simulink model "control"  (R2020b)
settings: Solver=VariableStepAuto  StartTime=0.0  StopTime=10.0  RelTol=1e-3
model workspace (MAT data in the model file):
  dt_planner = 0.01
undefined symbols (not defined in the file): DiscIntNeverNeededParam
settings Model: Creator=VVM  LastModifiedBy=VVM

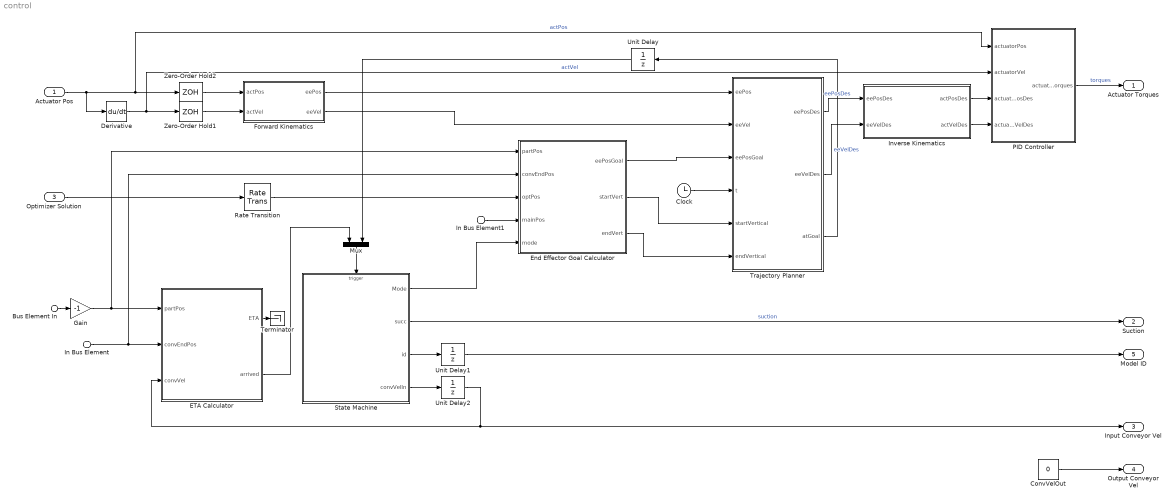
== system control ==
  Actuator Pos : Inport
  Bus Element In : Inport  Port=2  PortName=Camera Data  Element=model_position
  In Bus Element : Inport  Port=2  PortName=Camera Data  Element=beltEndPos
  In Bus Element1 : Inport  Port=2  PortName=Camera Data  Element=containerPos
  Optimizer Solution : Inport  Port=3
  Clock : Clock
  ConvVelOut : Constant  Value=0
  Derivative : Derivative  CoefficientInTFapproximation=0.0005
  ETA Calculator : MATLAB Function  TreatAsAtomicUnit=on
  End Effector Goal Calculator : MATLAB Function  TreatAsAtomicUnit=on
  Forward Kinematics : Subsystem
  Gain : Gain  Gain=-1
  Inverse Kinematics : Subsystem
  Mux : Mux  Inputs=2
  PID Controller : Subsystem  TreatAsAtomicUnit=on  mask(PID Controller){P=0.5, I=6, D=0.15}
  Rate Transition : RateTransition
  State Machine : Stateflow chart  TreatAsAtomicUnit=on
  Terminator : Terminator
  Trajectory Planner : MATLAB Function  TreatAsAtomicUnit=on
  Unit Delay : UnitDelay  SampleTime=-1  HasFrameUpgradeWarning=on
  Unit Delay1 : UnitDelay  InitialCondition=1  SampleTime=-1  HasFrameUpgradeWarning=on
  Unit Delay2 : UnitDelay  InitialCondition=1  SampleTime=-1  HasFrameUpgradeWarning=on
  Zero-Order Hold1 : ZeroOrderHold  SampleTime=-1
  Zero-Order Hold2 : ZeroOrderHold  SampleTime=-1
  Actuator Torques : Outport
  Suction : Outport  Port=2
  Input Conveyor Vel : Outport  Port=3
  Output Conveyor Vel : Outport  Port=4
  Model ID : Outport  Port=5
  wires:
  Optimizer Solution/1 -> Rate Transition/1
  State Machine/3(id) -> Unit Delay1/1
  Gain/1 -> End Effector Goal Calculator/1(partPos), ETA Calculator/1(partPos)
  ETA Calculator/1(ETA) -> Terminator/1
  Trajectory Planner/3(atGoal) -> Unit Delay/1
  Unit Delay1/1 -> Model ID/1
  Rate Transition/1 -> End Effector Goal Calculator/3(optPos)
  State Machine/2(succ) -> Suction/1  "suction"
  State Machine/1(Mode) -> End Effector Goal Calculator/5(mode)
  End Effector Goal Calculator/3(endVert) -> Trajectory Planner/6(endVertical)
  End Effector Goal Calculator/1(eePosGoal) -> Trajectory Planner/3(eePosGoal)
  End Effector Goal Calculator/2(startVert) -> Trajectory Planner/5(startVertical)
  Unit Delay2/1 -> Input Conveyor Vel/1, ETA Calculator/3(convVel)
  Mux/1 -> State Machine/Trigger
  Actuator Pos/1 -> Zero-Order Hold2/1, PID Controller/1(actuatorPos), Derivative/1  "actPos"
  State Machine/4(convVelIn) -> Unit Delay2/1
  Zero-Order Hold1/1 -> Forward Kinematics/2(actVel)
  Zero-Order Hold2/1 -> Forward Kinematics/1(actPos)
  Derivative/1 -> Zero-Order Hold1/1, PID Controller/2(actuatorVel)  "actVel"
  Inverse Kinematics/2(actVelDes) -> PID Controller/4(actuatorVelDes)
  Inverse Kinematics/1(actPosDes) -> PID Controller/3(actuatorPosDes)
  Unit Delay/1 -> Mux/2
  Trajectory Planner/1(eePosDes) -> Inverse Kinematics/1(eePosDes)  "eePosDes"
  ConvVelOut/1 -> Output Conveyor Vel/1
  In Bus Element/1 -> End Effector Goal Calculator/2(convEndPos), ETA Calculator/2(convEndPos)
  Forward Kinematics/2(eeVel) -> Trajectory Planner/2(eeVel)
  Clock/1 -> Trajectory Planner/4(t)
  Forward Kinematics/1(eePos) -> Trajectory Planner/1(eePos)
  PID Controller/1(actuatorTorques) -> Actuator Torques/1  "torques"
  Trajectory Planner/2(eeVelDes) -> Inverse Kinematics/2(eeVelDes)  "eeVelDes"
  ETA Calculator/2(arrived) -> Mux/1
  In Bus Element1/1 -> End Effector Goal Calculator/4(mainPos)
  Bus Element In/1 -> Gain/1

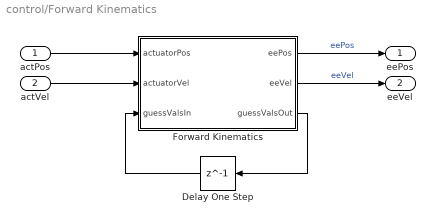
== system control/Forward Kinematics ==
  actPos : Inport
  actVel : Inport  Port=2
  Delay One Step : Delay  DelayLength=1
  Forward Kinematics : MATLAB Function  TreatAsAtomicUnit=on
  eePos : Outport
  eeVel : Outport  Port=2
  wires:
  Delay One Step/1 -> Forward Kinematics/3(guessValsIn)
  Forward Kinematics/3(guessValsOut) -> Delay One Step/1
  actPos/1 -> Forward Kinematics/1(actuatorPos)
  actVel/1 -> Forward Kinematics/2(actuatorVel)
  Forward Kinematics/1(eePos) -> eePos/1  "eePos"
  Forward Kinematics/2(eeVel) -> eeVel/1  "eeVel"

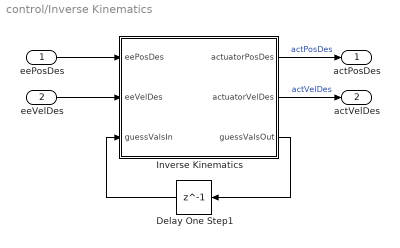
== system control/Inverse Kinematics ==
  eePosDes : Inport
  eeVelDes : Inport  Port=2
  Delay One Step1 : Delay  DelayLength=1
  Inverse Kinematics : MATLAB Function  TreatAsAtomicUnit=on
  actPosDes : Outport
  actVelDes : Outport  Port=2
  wires:
  Delay One Step1/1 -> Inverse Kinematics/3(guessValsIn)
  Inverse Kinematics/3(guessValsOut) -> Delay One Step1/1
  Inverse Kinematics/2(actuatorVelDes) -> actVelDes/1  "actVelDes"
  Inverse Kinematics/1(actuatorPosDes) -> actPosDes/1  "actPosDes"
  eeVelDes/1 -> Inverse Kinematics/2(eeVelDes)
  eePosDes/1 -> Inverse Kinematics/1(eePosDes)

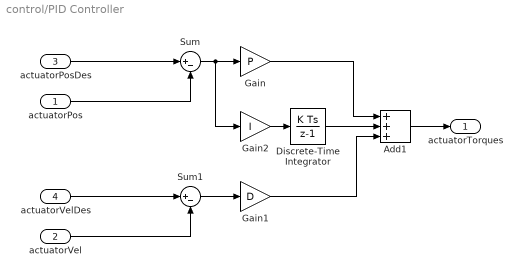
== system control/PID Controller ==
  actuatorPos : Inport
  actuatorVel : Inport  Port=2
  actuatorPosDes : Inport  Port=3
  actuatorVelDes : Inport  Port=4
  Add1 : Sum  Inputs=+++
  Discrete-Time Integrator : DiscreteIntegrator  gainval=1  SampleTime=-1  ICPrevOutput=DiscIntNeverNeededParam  ICPrevScaledInput=DiscIntNeverNeededParam
  Gain : Gain  Gain=P
  Gain1 : Gain  Gain=D
  Gain2 : Gain  Gain=I
  Sum : Sum  Inputs=|+-
  Sum1 : Sum  Inputs=|+-
  actuatorTorques : Outport
  wires:
  actuatorPosDes/1 -> Sum/1
  actuatorPos/1 -> Sum/2
  actuatorVel/1 -> Sum1/2
  Sum/1 -> Gain2/1, Gain/1
  Sum1/1 -> Gain1/1
  Gain/1 -> Add1/1
  Gain1/1 -> Add1/3
  Discrete-Time Integrator/1 -> Add1/2
  Gain2/1 -> Discrete-Time Integrator/1
  Add1/1 -> actuatorTorques/1
  actuatorVelDes/1 -> Sum1/1

== stateflow chart control/State Machine ==
  settings: executeAtInitialization=1
  state Hover
  state Grab
    entry:
    convVelIn = 0;
    exit:
    convVelIn = 1;
  state Retract2
  state Retract1
  state Drop
  note: Wait for object
      | to stabilize
  Hover -> Grab : arrived
  Grab -> Retract2 : atGoal
      | {succ = 1;}
  Retract1 -> Hover : atGoal
  Retract2 -> Drop : atGoal
  (default) -> Retract1
  (junction 406) -> Retract1 : after(15,msec)
      | {succ = 0; id = id + 1;}
  Drop -> (junction 406) : atGoal
  data: Mode output Enum: State; succ output; id output =1; convVelIn output =1
  events: arrived input RISING_EDGE_EVENT; atGoal input RISING_EDGE_EVENT

== matlab function control/Forward Kinematics/Forward Kinematics ==
  settings: updateMethod=DISCRETE  sampleTime=0.01
  data: actuatorPos input size=3; eePos output size=3; actuatorVel input size=3; guessValsIn input size=3; eeVel output; guessValsOut output size=3
function [eePos, eeVel, guessValsOut] = FK(actuatorPos, actuatorVel, guessValsIn)
% Wrapper around sm_pick_and_place_fk.m, which creates a persistent
% KinematicsSolver object for the forwards kinematics problem and then
% solves it.

coder.extrinsic('fk_solver');
persistent init
if isempty(init)
    init = true;
    eePos = zeros(3,1);
    eeVel = zeros(3,1);
    guessValsOut = zeros(3,1);
    status = 1;
end
[eePos, eeVel, guessValsOut, status] = fk_solver(actuatorPos, actuatorVel, guessValsIn);
if status ~= 1
    error('404 solution not found. Forward solve failed.')
end

== matlab function control/Inverse Kinematics/Inverse Kinematics ==
  settings: updateMethod=DISCRETE  sampleTime=0.01
  data: eePosDes input size=3; actuatorPosDes output size=3; eeVelDes input size=3; guessValsIn input size=3; actuatorVelDes output size=3; guessValsOut output size=3
function [actuatorPosDes, actuatorVelDes, guessValsOut] = IK(eePosDes, eeVelDes, guessValsIn)
% Wrapper around sm_pick_and_place_ik.m, which creates a persistent
% KinematicsSolver object for the inverse kinematics problem and then
% solves it.

coder.extrinsic('ik_solver');
persistent init
if isempty(init)
    init = true;
    actuatorPosDes = zeros(3,1);
    actuatorVelDes = zeros(3,1);
    guessValsOut = zeros(3,1);
    status = 1;
end
[actuatorPosDes, actuatorVelDes, guessValsOut, status] = ik_solver(eePosDes, eeVelDes, guessValsIn);
if status ~= 1
    error("Mathworks but your math doesn't. Inverse solve failed.");
end

== matlab function control/Trajectory Planner ==
  settings: updateMethod=DISCRETE
  data: eePos input size=3; eeVel input size=3; eePosGoal input size=3; eePosDes output size=3; t input size=1; startVertical input size=1; endVertical input size=1; eeVelDes output size=3; atGoal output
function [eePosDes, eeVelDes, atGoal] = gotoPosition(eePos, eeVel, eePosGoal, t, startVertical, endVertical)
% High-level function to go to a goal position.  Returns the desired
% position and and velocity at current time along the trajectory to a goal
% position. The time to goal along the trajectory is always set to 0.2
% seconds. startVertical and endVertical indicate whether the curve defined
% by the trajectory should begin and/or end vertically (i.e., the end
% effector should move straight up or down when starting or ending its
% motion).  It always assumed that the initial and final velocities and
% accelerations along the trajectory are zero.  Thus, the goal velocity is
% always zero. If the current position and velocity are sufficiently close
% to the goal position and velocity, 'done' is true.

persistent plan
if isempty(plan)
    plan = true;
end

if startVertical
    startDirectionGoal = [0;0;-0.2];
else
    startDirectionGoal = eeVel;
end
if endVertical
    endDirectionGoal = [0;0;0.2];
else
    endDirectionGoal = [0;0;0];
end
timeToGoal = 0.3;
[eePosDes, eeVelDes, atGoal] = gotoGoal(...
    plan, ...
    t, timeToGoal, ...
    eePos, eeVel, ...
    eePosGoal, startDirectionGoal, endDirectionGoal);
plan = atGoal;
end

function p = getPoly5(t0,tf,x0,v0,a0,xf,vf,af)
% Compute the 5th order polynomial 
% 
% poly(t) = a*t^5 + b*t^4 + c*t^3 + d*t^2 + e*t + f
%
% such that
%
% p(t0) = x0; p(tf) = xf
% p'(t0) = v0; p'(tf) = vf
% p''(to) = a0; p''(tf) = af
%
% Returns the coeffecient vector p = [a b c d e f]

A = [t0^5    t0^4    t0^3   t0^2 t0 1;
     5*t0^4  4*t0^3  3*t0^2 2*t0 1  0;
     20*t0^3 12*t0^2 6*t0   2    0  0;
     tf^5    tf^4    tf^3   tf^2 tf 1;
     5*tf^4  4*tf^3  3*tf^2 2*tf 1  0;
     20*tf^3 12*tf^2 6*tf   2    0  0];
b = [x0 v0 a0 xf vf af]';
p = A\b;
end

function p = getPoly3(t0,tf,x0,v0,xf,vf)
% Compute the 3rd order polynomial 
% 
% poly(t) = a*t^3 + b*t^2 + c*t + d
%
% such that
%
% p(t0) = x0; p(tf) = xf
% p'(t0) = v0; p'(tf) = vf
%
% Returns the coeffecient vector p = [a b c d]

A = [t0^3   t0^2 t0 1;
     3*t0^2 2*t0 1  0;
     tf^3   tf^2 tf 1;
     3*tf^2 2*tf 1  0];
b = [x0 v0 xf vf]';
p = A\b;
end

function [eePosDes, eeVelDes, atGoal] = gotoGoal(...
    plan, ...
    t, timeToGoal, ...
    eePos, eeVel, ...
    eePosGoal, startDirectionGoal, endDirectionGoal)
% Return desired position and and velocity at current time along the
% trajectory to a goal position.  The trajectory is only computed is 'plan'
% is true.  The trajectory is determined by the desired time to reach the
% goal (timeToGoal), the desired goal position (eePosGoal), and the
% starting and ending directions (startDirectionGoal and endDirectionGoal)
% of the curve to the goal in xyz camera coordinates.  It always assumed
% that the initial and final velocities and accelerations along the
% trajectory are zero.  Thus, the goal velocity is always zero.  If the
% current position and velocity are sufficiently close to the goal position
% and velocity, 'atGoal' is true.

persistent cpoly cdpoly spoly sdpoly t0 tf ...
    maxErrPos maxErrVel

if isempty(tf)
    cpoly = zeros(3,4);
    cdpoly = zeros(3,3);
    spoly = zeros(1,6);
    sdpoly = zeros(1,5);
    
    t0 = t;
    tf = t;
    
    maxErrPos = 0.02;
    maxErrVel = 0.1;
end

errPos = eePosGoal - eePos;
errVel = -eeVel;
errPosNorm = norm(errPos);
errVelNorm = norm(errVel);

if plan
    t0 = t;
    tf = t0 + timeToGoal;
    [cpoly, cdpoly, spoly, sdpoly] = getTrajectory(...
        t0, tf, eePos, eePosGoal, startDirectionGoal, endDirectionGoal);
end

t = min(t,tf); %if t > tf, we just want to keep aiming for end of trajectory
s = polyval(spoly,t);
eePosDes = [polyval(cpoly(1,:),s);polyval(cpoly(2,:),s);polyval(cpoly(3,:),s)];
eeVelDes = [polyval(cdpoly(1,:),s);polyval(cdpoly(2,:),s);polyval(cdpoly(3,:),s)]*polyval(sdpoly,t);
atGoal = errPosNorm < maxErrPos && errVelNorm < maxErrVel;
end

function [cpoly, cdpoly, spoly, sdpoly] = getTrajectory(...
    t0, tf, eePos, eePosGoal, startDirectionGoal, endDirectionGoal)
% Return polynomials needed to compute a time-scaled trajectory
% from eePos to eePosGoal such that initial and final velocities
% and accelerations are zero.  The path of the trajectory in xyz space has
% an initial tangent equal to startDirectionGoal and an ending tangent of
% endDirectionGoal.
%
% Let c(s) = [x(s);y(s);z(s)] with s = [0 1] be a curve in xyz space from
% eePos to eePosGoal.  We assume each element is a 3rd order
% polymonial and compute the corresponding 3-by-4 coefficient matrix,
% cpoly:
%
%         [a1*s^3 + b1*s^2 + c1*s + d1]           [s^3]
%  c(s) = [a2*s^3 + b2*s^2 + c2*s + d2] = cpoly * [s^2]
%         [a3*s^3 + b3*s^2 + c3*s + d3]           [s  ]
%                                                 [1  ]
%
% The 12 coefficeints in cpoly are uniquely determined by the following
% boundary conditions:
%
% c(0) = eePos
% c(1) = eePosGoal
% c'(0) = startDirectionGoal
% c'(1) = endDirectionGoal
%
% cdpoly is a 3-by-3 matrix of polynomial coefficents of the derivatives of
% each row of cpoly:
%
%          [3*a1 2*b1 c1]
% cdpoly = [3*a2 2*b2 c2]
%          [3*a3 2*b3 c3]
%
% The curve c(s) is then time-scaled to ensure that the initial and final
% speeds and accelerations along the curve are zero.  The time scaling
% s(t) is a 5th order polynomial
%
%  s(t) = A*s^5 + B*s^4 + C*s^3 + D*s^2 + E*s + F
%
%       = spoly*[s^5 s^4 s^3 s^2 s 1]'
%
% spoly is a 1-by-6 vector of coefficents with values uniquely determined
% by the following boundary conditions:
%
% s(t0) = 0
% s(tf) = 1
% s'(t0) = 0
% s'(tf) = 0
% s''(t0) = 0
% s''(tf) = 0
%
% sdpoly is a 1-by-5 matrix of polynomial coefficents of the derivative of
% spoly:
%
% sdpoly = [5*A 4*B 3*C 2*D E]
%
% The final time-scaled trajectory corresponds to c(s(t))

s0 = 0;
sf = 1;
c0 = eePos;
cf = eePosGoal;
cd0 = startDirectionGoal;
cdf = endDirectionGoal;
cpoly = zeros(3,4);
cdpoly = zeros(3,3);
for i = 1:3
    cpoly(i,:) = getPoly3(s0,sf,c0(i),cd0(i),cf(i),cdf(i));
    % Need to be careful with polyder.  If the polynomial is equivalent
    % to just a constant (e.g., [0 0 0 1]), then polyder returns [0]
    % instead of [0 0 0].
    pd = polyder(cpoly(i,:));
    if length(pd) == 3
        cdpoly(i,:) = pd;
    else
        cdpoly(i,:) = [0 0 0];
    end
end

s0 = 0;
sf = 1;
sd0 = 0;
sdf = 0;
sdd0 = 0;
sddf = 0;
spoly = getPoly5(t0,tf,s0,sd0,sdd0,sf,sdf,sddf);
sdpoly = polyder(spoly);
end

== matlab function control/ETA Calculator ==
  data: partPos input; ETA output; convEndPos input; convVel input; arrived output
function [ETA, arrived] = Calculator(partPos, convEndPos, convVel)
    dist = partPos(1:2) - convEndPos(1:2);
    ETA = norm(dist) / convVel;
    arrived = (ETA <= 0.05);
end

== matlab function control/End Effector Goal Calculator ==
  data: eePosGoal output size=3; startVert output; partPos input; convEndPos input; endVert output; optPos input; mainPos input; mode input
function [eePosGoal, startVert, endVert] = Planner(partPos, convEndPos, optPos, mainPos, mode)

switch mode
    case State.Grab
        % Pick up object
        eePosGoal = partPos;
        startVert = false;
        endVert = true;
        
    case State.Retract1
        % Hover above container
        eePosGoal = mainPos;
        startVert = false;
        endVert = false;
        
    case State.Retract2
        % Hover even higher above container
        eePosGoal = mainPos - [0; 0; 0.04];
        startVert = true;
        endVert = true;
        
    case State.Drop
        % Drop object
        eePosGoal = optPos;
        startVert = false;
        endVert = true;
        
    case State.Hover
        % Hover above conveyor
        eePosGoal = convEndPos - [0; 0; 0.1];
        startVert = false;
        endVert = false;
        
    otherwise
        error('invalid mode')
end
end
